simulink model "V90_2MW_TurbineModel_26_11_2021"  (R2020a)
settings: Solver=VariableStepAuto  StartTime=0.0  StopTime=10  RelTol=1e-3  EnableMultiTasking=on
model workspace (MAT data in the model file):
  Tw = Simulink.Parameter
  Tw.Value = [0; 0; 24.07; 18.74; 14.42; 10.93; 8.08; 5.74; 5.8; 4.17; 2.78; 1.59; 0.56; -0.34; -1.13; -1.83; -2.46; -3.02; -3.52; -3.98; -4.39; -3.77; -4.12; -4.43; -4.73]
  Tw.DataType = 'auto'
  Tw.Dimensions = [25 1]
  c = Simulink.Parameter
  c.Value = [3.65; 4.43; 4.56; 4.36; 4.03; 3.68; 3.35; 3.05; 2.79; 2.56; 2.37; 2.19; 2.04; 1.91; 1.79; 1.68; 1.59; 1.5; 1.43; 1.36; 1.29; 1.24; 1.18; 1.14; 1.09]
  c.DataType = 'auto'
  c.Dimensions = [25 1]
  dcm = Simulink.Parameter
  dcm.Value = [0  0  0; 0  0  0; 0  0  0]
  dcm.DataType = 'auto'
  dcm.Dimensions = [3 3]
  r = Simulink.Parameter
  r.Value = [1.8; 3.6; 5.4; 7.2; 9; 10.8; 12.6; 14.4; 16.2; 18; 19.8; 21.6; 23.4; 25.2; 27; 28.8; 30.6; 32.4; 34.2; 36; 37.8; 39.6; 41.4; 43.2; 45]
  r.DataType = 'auto'
  r.Dimensions = [25 1]
values from neighbouring files (symbols this model uses):
  N = 100    [Generator_specs.m]
  s = tf('s')    [Wind_Turbine_Pitch.m]
undefined symbols (not defined in the file or in its folder): T, X, Y, Z
libraries: sm_lib x21, nesl_utility x12, fl_lib x5, aerolibtransform2 x3, aerolibwind2 x3, aerolib6dof2 x1, simulink x1, aerolibasang x1
(part 1 of 2)
settings Model: Creator=Dimple  LastModifiedBy=Dimple
settings DataIOCC: LimitDataPoints=on  MaxDataPoints=10000
settings OptimizationCC: LifeSpan=inf
settings DebuggingCC: AllowSymbolicDim=off  SFUnexpectedBacktrackingDiag=warning  SFNoUnconditionalDefaultTransitionDiag=warning  SFExecutionAtInitializationDiag=none  ArithmeticOperatorsInVariantConditions=warning
settings SFSimCC: SimUseLocalCustomCode=off  CustomCodeUndefinedFunction=UseInterfaceOnly
settings RTWCC: RTWUseLocalCustomCode=off
settings CodeAppCC: StateflowObjectComments=on
settings GRTTargetCC: TargetLangStandard=C89/C90 (ANSI)
settings ConfigComp: CovMetricSettings=dw  CovHtmlReporting=on  CovSaveCumulativeToWorkspaceVar=on  CovSaveSingleToWorkspaceVar=on  CovExternalEMLEnable=off  CovSFcnEnable=off
settings SimscapeCC: SimscapeLogType=all  SimscapeLogSimulationStatistics=on  SimscapeLogDataHistory=10000

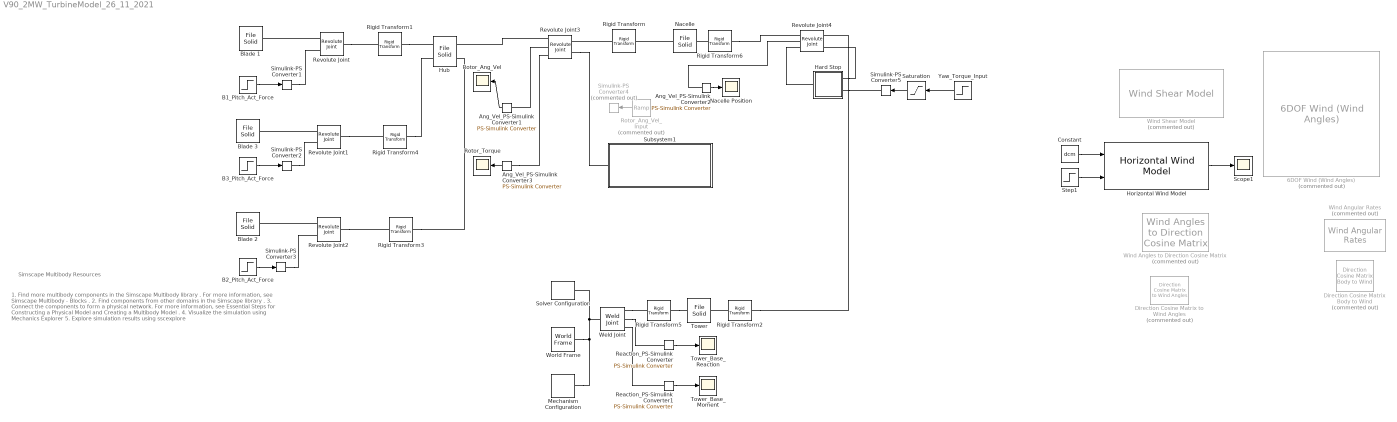
== system V90_2MW_TurbineModel_26_11_2021 ==
  note: 1. Find more multibody components in the Simscape Multibody library .
      | For more information, see Simscape Multibody - Blocks .
      | 2. Find components from other domains in the Simscape library .
      | 3. Connect the components to form a physical network.
      | For more information, see Essential Steps for Constructing a Physical Model and Creating a Multibody Model .
      | 4. Visualize the simulation using Mechanics Explorer
      | 5. Explore simulation results using sscexplore
  note: Simscape Multibody Resources
  6DOF Wind (Wind Angles) : aerolib6dof2/6DOF Wind (Wind Angles)  Commented=on  units=Metric (MKS)  mtype=Fixed  rep=Wind Angles  xme_0=[0 0 0]  Vm_0=[0 0 0]  wind_0=[0 0 0]  pm_0=[0 0 0]  mass_0=1.0  mass_e=0.5  mass_f=2.0  inertia=eye(3)  inertia_e=eye(3)  inertia_f=2*eye(3)  vre_flag=on  abi_flag=off  xme_statename=''  Vm_statename=''  alpha_statename=''  beta_statename=''  wind_statename=''  quat_statename=''  pm_statename=''  mass_statename=''
      settings: SourceProductBaseCode=AE
  Ang_Vel_PS-Simulink Converter1 : nesl_utility/PS-Simulink Converter  PhysicalDomain=network_engine_domain  SubClassName=ps_output  LeftPortType=input  RightPortType=output  PseudoPeriodic=off  Frequencies=[]  Unit=inherit  AffineConversion=off
      settings: SourceProductBaseCode=MT,SS
  Ang_Vel_PS-Simulink Converter2 : nesl_utility/PS-Simulink Converter  PhysicalDomain=network_engine_domain  SubClassName=ps_output  LeftPortType=input  RightPortType=output  PseudoPeriodic=off  Frequencies=[]  Unit=inherit  AffineConversion=off
      settings: SourceProductBaseCode=MT,SS
  Ang_Vel_PS-Simulink Converter3 : nesl_utility/PS-Simulink Converter  PhysicalDomain=network_engine_domain  SubClassName=ps_output  LeftPortType=input  RightPortType=output  PseudoPeriodic=off  Frequencies=[]  Unit=inherit  AffineConversion=off
      settings: SourceProductBaseCode=MT,SS
  B1_Pitch_Act_Force : Step  Time=0.35  After=2  SampleTime=0
  B2_Pitch_Act_Force : Step  Time=0.35  After=2  SampleTime=0
  B3_Pitch_Act_Force : Step  Time=0.35  After=2  SampleTime=0
  Blade 1 : sm_lib/Body Elements/File Solid  ExtGeomFileName=C:\Users\Dimple\Desktop\Dimple\08_ALTRAN\01_Work\Wind Turbine_MBSE Design\01_WT_MBSE\Multibody\WT blade.STEP  UnitType=FromFile  ExtGeomFileUnits=m  StepReaderType=HEX  ExportConvexHullGeometry=off  InertiaType=PointMass  Mass=5388  MassUnits=kg  CenterOfMass=[0 0 0]  CenterOfMassUnits=m  MomentsOfInertia=[1 1 1]  MomentsOfInertiaUnits=kg*m^2  ProductsOfInertia=[0 0 0]  ProductsOfInertiaUnits=kg*m^2  BasedOnType=DensityFromFile  Density=1000  DensityUnits=kg/m^3  DoExposeReferenceFrame=on  SerializedFrames=<Frames/>  GraphicType=FromGeometry  MarkerShape=Sphere  MarkerSize=10  GraphicVisPropType=SimpleVisualProperties  GraphicDiffuseColor=[0.5 0.5 0.5]  GraphicSpecularColor=[0.5 0.5 0.5 1.0]  GraphicAmbientColor=[0.15 0.15 0.15 1.0]  GraphicEmissiveColor=[0.0 0.0 0.0 1.0]  GraphicShininess=75  GraphicOpacity=1.0
  Blade 2 : sm_lib/Body Elements/File Solid  ExtGeomFileName=C:\Users\Dimple\Desktop\Dimple\08_ALTRAN\01_Work\Wind Turbine_MBSE Design\01_WT_MBSE\Multibody\WT blade.STEP  UnitType=FromFile  ExtGeomFileUnits=m  StepReaderType=HEX  ExportConvexHullGeometry=off  InertiaType=PointMass  Mass=5388  MassUnits=kg  CenterOfMass=[0 0 0]  CenterOfMassUnits=m  MomentsOfInertia=[1 1 1]  MomentsOfInertiaUnits=kg*m^2  ProductsOfInertia=[0 0 0]  ProductsOfInertiaUnits=kg*m^2  BasedOnType=DensityFromFile  Density=1000  DensityUnits=kg/m^3  DoExposeReferenceFrame=on  SerializedFrames=<Frames/>  GraphicType=FromGeometry  MarkerShape=Sphere  MarkerSize=10  GraphicVisPropType=SimpleVisualProperties  GraphicDiffuseColor=[0.5 0.5 0.5]  GraphicSpecularColor=[0.5 0.5 0.5 1.0]  GraphicAmbientColor=[0.15 0.15 0.15 1.0]  GraphicEmissiveColor=[0.0 0.0 0.0 1.0]  GraphicShininess=75  GraphicOpacity=1.0
  Blade 3 : sm_lib/Body Elements/File Solid  ExtGeomFileName=C:\Users\Dimple\Desktop\Dimple\08_ALTRAN\01_Work\Wind Turbine_MBSE Design\01_WT_MBSE\Multibody\WT blade.STEP  UnitType=FromFile  ExtGeomFileUnits=m  StepReaderType=HEX  ExportConvexHullGeometry=off  InertiaType=PointMass  Mass=5388  MassUnits=kg  CenterOfMass=[0 0 0]  CenterOfMassUnits=m  MomentsOfInertia=[1 1 1]  MomentsOfInertiaUnits=kg*m^2  ProductsOfInertia=[0 0 0]  ProductsOfInertiaUnits=kg*m^2  BasedOnType=DensityFromFile  Density=1000  DensityUnits=kg/m^3  DoExposeReferenceFrame=on  SerializedFrames=<Frames/>  GraphicType=FromGeometry  MarkerShape=Sphere  MarkerSize=10  GraphicVisPropType=SimpleVisualProperties  GraphicDiffuseColor=[0.5 0.5 0.5]  GraphicSpecularColor=[0.5 0.5 0.5 1.0]  GraphicAmbientColor=[0.15 0.15 0.15 1.0]  GraphicEmissiveColor=[0.0 0.0 0.0 1.0]  GraphicShininess=75  GraphicOpacity=1.0
  Constant : Constant  Value=dcm
  Direction Cosine Matrix Body to Wind : aerolibtransform2/Direction Cosine Matrix Body to Wind  Commented=on
      settings: SourceProductBaseCode=AE
  Direction Cosine Matrix to Wind Angles : aerolibtransform2/Direction Cosine Matrix to Wind Angles  Commented=on  action=None  tolerance=eps(2)
      settings: SourceProductBaseCode=AE
  Hard Stop : Subsystem  mask{ub=pi()/4, lb=0, csub=1e+04, cslb=1e+06, cdub=1e7, cdlb=1e7, iap=0}
      mask prompts: ub "Upper bound (rad)"; lb "Lower bound (rad)"; csub "Contact stiffness at upper bound (N*m/rad)"; cslb "Contact stiffness at lower bound (N*m/rad)"; cdub "Contact damping at upper bound (N*m/(rad/s))"; cdlb "Contact damping at lower bound (N*m/(rad/s))"; iap "Initial angular position"
      mask Display: image(imread('Hard Stop.png'))
  Horizontal Wind Model : aerolibwind2/Horizontal Wind Model  units=Metric (MKS)  Vw_source=External  Vwind=13.5  W_source=Internal  Wdeg=30
      settings: SourceProductBaseCode=AE
  Hub : sm_lib/Body Elements/File Solid  ExtGeomFileName=C:\Users\Dimple\Desktop\Dimple\08_ALTRAN\01_Work\Wind Turbine_MBSE Design\01_WT_MBSE\Multibody\WT hub.STEP  UnitType=FromFile  ExtGeomFileUnits=m  StepReaderType=HEX  ExportConvexHullGeometry=off  InertiaType=PointMass  Mass=18770  MassUnits=kg  CenterOfMass=[0 0 0]  CenterOfMassUnits=m  MomentsOfInertia=[1 1 1]  MomentsOfInertiaUnits=kg*m^2  ProductsOfInertia=[0 0 0]  ProductsOfInertiaUnits=kg*m^2  BasedOnType=DensityFromFile  Density=1000  DensityUnits=kg/m^3  DoExposeReferenceFrame=on  SerializedFrames=<Frames><Frame><Id>Frame1</Id><Value><Name>B1</Name><Origin><Source>GeometricFeature</Source><FeatureName>circular curve 23</FeatureName></Origin><PrimaryAxis><DefinedDirection>+Z</DefinedDirection><Source>ReferenceFrame</Source><SourceDirection>+Y</SourceDirection><FeatureName></FeatureName></PrimaryAxis><SecondaryAxis><DefinedDirection>+X</DefinedDirection><Source>ReferenceFrame</Source><SourceDirection>+X</SourceDirection><FeatureName></FeatureName></SecondaryAxis></Value></Frame><Frame><Id>Frame3</Id><Value><Name>B3</Name><Origin><Source>GeometricFeature</Source><FeatureName>circular curve 21</FeatureName></Origin><PrimaryAxis><DefinedDirection>+Z</DefinedDirection><Source>ReferenceFrame</Source><SourceDirection>-X</SourceDirection><FeatureName></FeatureName></PrimaryAxis><SecondaryAxis><DefinedDirection>+X</DefinedDirection><Source>ReferenceFrame</Source><SourceDirection>-Y</SourceDirection><FeatureName></FeatureName></SecondaryAxis></Value></Frame><Frame><Id>Frame4</Id><Value><Name>B2</Name><Origin><Source>GeometricFeature</Source><FeatureName>circular curve 25</FeatureName></Origin><PrimaryAxis><DefinedDirection>+Z</DefinedDirection><Source>ReferenceFrame</Source><SourceDirection>+X</SourceDirection><FeatureName></FeatureName></PrimaryAxis><SecondaryAxis><DefinedDirection>+X</DefinedDirection><Source>ReferenceFrame</Source><SourceDirection>+Y</SourceDirection><FeatureName></FeatureName></SecondaryAxis></Value></Frame></Frames>  GraphicType=FromGeometry  MarkerShape=Sphere  MarkerSize=10  GraphicVisPropType=SimpleVisualProperties  GraphicDiffuseColor=[0.5 0.5 0.5]  GraphicSpecularColor=[0.5 0.5 0.5 1.0]  GraphicAmbientColor=[0.15 0.15 0.15 1.0]  GraphicEmissiveColor=[0.0 0.0 0.0 1.0]  GraphicShininess=75  GraphicOpacity=1.0
  Mechanism Configuration : sm_lib/Utilities/Mechanism Configuration  UniformGravity=Constant  GravityVector=[0 -9.80665 0]  GravityUnits=m/s^2  LinearizationDelta=0.001
  Nacelle : sm_lib/Body Elements/File Solid  ExtGeomFileName=C:\Users\Dimple\Desktop\Dimple\08_ALTRAN\01_Work\Wind Turbine_MBSE Design\01_WT_MBSE\Multibody\WT nacelle.STEP  UnitType=FromFile  ExtGeomFileUnits=m  StepReaderType=HEX  ExportConvexHullGeometry=off  InertiaType=PointMass  Mass=56310  MassUnits=kg  CenterOfMass=[0 0 0]  CenterOfMassUnits=m  MomentsOfInertia=[1 1 1]  MomentsOfInertiaUnits=kg*m^2  ProductsOfInertia=[0 0 0]  ProductsOfInertiaUnits=kg*m^2  BasedOnType=DensityFromFile  Density=1000  DensityUnits=kg/m^3  DoExposeReferenceFrame=on  SerializedFrames=<Frames><Frame><Id>Frame1</Id><Value><Name>T</Name><Origin><Source>GeometricFeature</Source><FeatureName>circular curve 2</FeatureName></Origin><PrimaryAxis><DefinedDirection>+Z</DefinedDirection><Source>ReferenceFrame</Source><SourceDirection>+Z</SourceDirection><FeatureName></FeatureName></PrimaryAxis><SecondaryAxis><DefinedDirection>+X</DefinedDirection><Source>ReferenceFrame</Source><SourceDirection>+X</SourceDirection><FeatureName></FeatureName></SecondaryAxis></Value></Frame></Frames>  GraphicType=FromGeometry  MarkerShape=Sphere  MarkerSize=10  GraphicVisPropType=SimpleVisualProperties  GraphicDiffuseColor=[0.5 0.5 0.5]  GraphicSpecularColor=[0.5 0.5 0.5 1.0]  GraphicAmbientColor=[0.15 0.15 0.15 1.0]  GraphicEmissiveColor=[0.0 0.0 0.0 1.0]  GraphicShininess=75  GraphicOpacity=1.0
  Nacelle Position : Scope
  Reaction_PS-Simulink Converter : nesl_utility/PS-Simulink Converter  PhysicalDomain=network_engine_domain  SubClassName=ps_output  LeftPortType=input  RightPortType=output  PseudoPeriodic=off  Frequencies=[]  Unit=inherit  AffineConversion=off
      settings: SourceProductBaseCode=MT,SS
  Reaction_PS-Simulink Converter1 : nesl_utility/PS-Simulink Converter  PhysicalDomain=network_engine_domain  SubClassName=ps_output  LeftPortType=input  RightPortType=output  PseudoPeriodic=off  Frequencies=[]  Unit=inherit  AffineConversion=off
      settings: SourceProductBaseCode=MT,SS
  Revolute Joint : sm_lib/Joints/Revolute Joint  JointMode=Normal  SenseConstraintForce=off  SenseConstraintForceX=off  SenseConstraintForceY=off  SenseConstraintForceZ=off  SenseConstraintTorque=off  SenseConstraintTorqueX=off  SenseConstraintTorqueY=off  SenseConstraintTorqueZ=off  SenseTotalForce=off  SenseTotalForceX=off  SenseTotalForceY=off  SenseTotalForceZ=off  SenseTotalTorque=off  SenseTotalTorqueX=off  SenseTotalTorqueY=off  SenseTotalTorqueZ=off  CompositeWrenchDir=BaseOnFollower  CompositeWrenchFrame=BaseFrame  EquilibriumPosition=0  EquilibriumPositionUnits=deg  SpringStiffness=0  SpringStiffnessUnits=N*m/deg  DampingCoefficient=0  DampingCoefficientUnits=N*m/(deg/s)  TorqueActuationMode=ComputedTorque  MotionActuationMode=InputMotion  SensePosition=off  SenseVelocity=off  SenseAcceleration=off  SenseTorqueForce=off  SenseLowerLimitTorqueForce=off  SenseUpperLimitTorqueForce=off  LowerLimitSpecify=off  LowerLimitBound=-90  LowerLimitBoundUnits=deg  LowerLimitStiffness=1e4  LowerLimitStiffnessUnits=N*m/deg  LowerLimitDamping=10  LowerLimitDampingUnits=N*m/(deg/s)  LowerLimitTransitionRegionWidth=0.1  LowerLimitTransitionRegionWidthUnits=deg  UpperLimitSpecify=off  UpperLimitBound=90  UpperLimitBoundUnits=deg  UpperLimitStiffness=1e4  UpperLimitStiffnessUnits=N*m/deg  UpperLimitDamping=10  UpperLimitDampingUnits=N*m/(deg/s)  UpperLimitTransitionRegionWidth=0.1  UpperLimitTransitionRegionWidthUnits=deg  PositionTargetSpecify=off  PositionTargetPriority=High  PositionTargetValue=30  PositionTargetValueUnits=deg  VelocityTargetSpecify=off  VelocityTargetPriority=High  VelocityTargetValue=0  VelocityTargetValueUnits=deg/s
  Revolute Joint1 : sm_lib/Joints/Revolute Joint  JointMode=Normal  SenseConstraintForce=off  SenseConstraintForceX=off  SenseConstraintForceY=off  SenseConstraintForceZ=off  SenseConstraintTorque=off  SenseConstraintTorqueX=off  SenseConstraintTorqueY=off  SenseConstraintTorqueZ=off  SenseTotalForce=off  SenseTotalForceX=off  SenseTotalForceY=off  SenseTotalForceZ=off  SenseTotalTorque=off  SenseTotalTorqueX=off  SenseTotalTorqueY=off  SenseTotalTorqueZ=off  CompositeWrenchDir=BaseOnFollower  CompositeWrenchFrame=BaseFrame  EquilibriumPosition=0  EquilibriumPositionUnits=deg  SpringStiffness=0  SpringStiffnessUnits=N*m/deg  DampingCoefficient=0  DampingCoefficientUnits=N*m/(deg/s)  TorqueActuationMode=ComputedTorque  MotionActuationMode=InputMotion  SensePosition=off  SenseVelocity=off  SenseAcceleration=off  SenseTorqueForce=off  SenseLowerLimitTorqueForce=off  SenseUpperLimitTorqueForce=off  LowerLimitSpecify=off  LowerLimitBound=-90  LowerLimitBoundUnits=deg  LowerLimitStiffness=1e4  LowerLimitStiffnessUnits=N*m/deg  LowerLimitDamping=10  LowerLimitDampingUnits=N*m/(deg/s)  LowerLimitTransitionRegionWidth=0.1  LowerLimitTransitionRegionWidthUnits=deg  UpperLimitSpecify=off  UpperLimitBound=90  UpperLimitBoundUnits=deg  UpperLimitStiffness=1e4  UpperLimitStiffnessUnits=N*m/deg  UpperLimitDamping=10  UpperLimitDampingUnits=N*m/(deg/s)  UpperLimitTransitionRegionWidth=0.1  UpperLimitTransitionRegionWidthUnits=deg  PositionTargetSpecify=off  PositionTargetPriority=High  PositionTargetValue=30  PositionTargetValueUnits=deg  VelocityTargetSpecify=off  VelocityTargetPriority=High  VelocityTargetValue=0  VelocityTargetValueUnits=deg/s
  Revolute Joint2 : sm_lib/Joints/Revolute Joint  JointMode=Normal  SenseConstraintForce=off  SenseConstraintForceX=off  SenseConstraintForceY=off  SenseConstraintForceZ=off  SenseConstraintTorque=off  SenseConstraintTorqueX=off  SenseConstraintTorqueY=off  SenseConstraintTorqueZ=off  SenseTotalForce=off  SenseTotalForceX=off  SenseTotalForceY=off  SenseTotalForceZ=off  SenseTotalTorque=off  SenseTotalTorqueX=off  SenseTotalTorqueY=off  SenseTotalTorqueZ=off  CompositeWrenchDir=BaseOnFollower  CompositeWrenchFrame=BaseFrame  EquilibriumPosition=0  EquilibriumPositionUnits=deg  SpringStiffness=0  SpringStiffnessUnits=N*m/deg  DampingCoefficient=0  DampingCoefficientUnits=N*m/(deg/s)  TorqueActuationMode=ComputedTorque  MotionActuationMode=InputMotion  SensePosition=off  SenseVelocity=off  SenseAcceleration=off  SenseTorqueForce=off  SenseLowerLimitTorqueForce=off  SenseUpperLimitTorqueForce=off  LowerLimitSpecify=off  LowerLimitBound=-90  LowerLimitBoundUnits=deg  LowerLimitStiffness=1e4  LowerLimitStiffnessUnits=N*m/deg  LowerLimitDamping=10  LowerLimitDampingUnits=N*m/(deg/s)  LowerLimitTransitionRegionWidth=0.1  LowerLimitTransitionRegionWidthUnits=deg  UpperLimitSpecify=off  UpperLimitBound=90  UpperLimitBoundUnits=deg  UpperLimitStiffness=1e4  UpperLimitStiffnessUnits=N*m/deg  UpperLimitDamping=10  UpperLimitDampingUnits=N*m/(deg/s)  UpperLimitTransitionRegionWidth=0.1  UpperLimitTransitionRegionWidthUnits=deg  PositionTargetSpecify=off  PositionTargetPriority=High  PositionTargetValue=30  PositionTargetValueUnits=deg  VelocityTargetSpecify=off  VelocityTargetPriority=High  VelocityTargetValue=0  VelocityTargetValueUnits=deg/s
  Revolute Joint3 : sm_lib/Joints/Revolute Joint  JointMode=Normal  SenseConstraintForce=off  SenseConstraintForceX=off  SenseConstraintForceY=off  SenseConstraintForceZ=off  SenseConstraintTorque=off  SenseConstraintTorqueX=off  SenseConstraintTorqueY=off  SenseConstraintTorqueZ=off  SenseTotalForce=off  SenseTotalForceX=off  SenseTotalForceY=off  SenseTotalForceZ=off  SenseTotalTorque=off  SenseTotalTorqueX=off  SenseTotalTorqueY=off  SenseTotalTorqueZ=off  CompositeWrenchDir=FollowerOnBase  CompositeWrenchFrame=BaseFrame  EquilibriumPosition=0  EquilibriumPositionUnits=deg  SpringStiffness=0  SpringStiffnessUnits=N*m/deg  DampingCoefficient=0  DampingCoefficientUnits=N*m/(deg/s)  TorqueActuationMode=InputTorque  MotionActuationMode=ComputedMotion  SensePosition=off  SenseVelocity=on  SenseAcceleration=off  SenseTorqueForce=on  SenseLowerLimitTorqueForce=off  SenseUpperLimitTorqueForce=off  LowerLimitSpecify=off  LowerLimitBound=-90  LowerLimitBoundUnits=deg  LowerLimitStiffness=1e4  LowerLimitStiffnessUnits=N*m/deg  LowerLimitDamping=10  LowerLimitDampingUnits=N*m/(deg/s)  LowerLimitTransitionRegionWidth=0.1  LowerLimitTransitionRegionWidthUnits=deg  UpperLimitSpecify=off  UpperLimitBound=90  UpperLimitBoundUnits=deg  UpperLimitStiffness=1e4  UpperLimitStiffnessUnits=N*m/deg  UpperLimitDamping=10  UpperLimitDampingUnits=N*m/(deg/s)  UpperLimitTransitionRegionWidth=0.1  UpperLimitTransitionRegionWidthUnits=deg  PositionTargetSpecify=off  PositionTargetPriority=High  PositionTargetValue=0  PositionTargetValueUnits=deg  VelocityTargetSpecify=off  VelocityTargetPriority=High  VelocityTargetValue=0  VelocityTargetValueUnits=deg/s
  Revolute Joint4 : sm_lib/Joints/Revolute Joint  JointMode=Normal  SenseConstraintForce=off  SenseConstraintForceX=off  SenseConstraintForceY=off  SenseConstraintForceZ=off  SenseConstraintTorque=off  SenseConstraintTorqueX=off  SenseConstraintTorqueY=off  SenseConstraintTorqueZ=off  SenseTotalForce=off  SenseTotalForceX=off  SenseTotalForceY=off  SenseTotalForceZ=off  SenseTotalTorque=off  SenseTotalTorqueX=off  SenseTotalTorqueY=off  SenseTotalTorqueZ=off  CompositeWrenchDir=FollowerOnBase  CompositeWrenchFrame=BaseFrame  EquilibriumPosition=0  EquilibriumPositionUnits=deg  SpringStiffness=0  SpringStiffnessUnits=N*m/deg  DampingCoefficient=0  DampingCoefficientUnits=N*m/(deg/s)  TorqueActuationMode=InputTorque  MotionActuationMode=ComputedMotion  SensePosition=on  SenseVelocity=on  SenseAcceleration=off  SenseTorqueForce=off  SenseLowerLimitTorqueForce=off  SenseUpperLimitTorqueForce=off  LowerLimitSpecify=off  LowerLimitBound=0  LowerLimitBoundUnits=deg  LowerLimitStiffness=1e4  LowerLimitStiffnessUnits=N*m/deg  LowerLimitDamping=10  LowerLimitDampingUnits=N*m/(deg/s)  LowerLimitTransitionRegionWidth=0.1  LowerLimitTransitionRegionWidthUnits=deg  UpperLimitSpecify=off  UpperLimitBound=120  UpperLimitBoundUnits=deg  UpperLimitStiffness=1e4  UpperLimitStiffnessUnits=N*m/deg  UpperLimitDamping=10  UpperLimitDampingUnits=N*m/(deg/s)  UpperLimitTransitionRegionWidth=0.1  UpperLimitTransitionRegionWidthUnits=deg  PositionTargetSpecify=off  PositionTargetPriority=High  PositionTargetValue=30  PositionTargetValueUnits=deg  VelocityTargetSpecify=off  VelocityTargetPriority=High  VelocityTargetValue=0  VelocityTargetValueUnits=deg/s
  Rigid Transform : sm_lib/Frames and Transforms/Rigid Transform  TranslationMethod=StandardAxis  TranslationStandardOffset=4.5  TranslationLengthUnit=m  TranslationStandardAxis=+Z  TranslationCartesianOffset=[0 0 0]  TranslationROffset=0  TranslationROffsetUnits=m  TranslationZOffset=0  TranslationZOffsetUnits=m  TranslationThetaOffset=0  TranslationThetaOffsetUnits=deg  RotationMethod=None  RotationAngleUnits=deg  RotationStandardAxis=+Z  RotationAngle=0.0  RotationArbitraryAxis=[0 0 1]  FollAlignAxisA=+X  BaseAlignAxisA=+Y  FollAlignAxisB=+Y  BaseAlignAxisB=+Z  RotationSequenceAxes=FollowerAxes  RotationSequence=XYX  RotationSequenceAngles=[0 0 0]  RotationSequenceAnglesUnits=deg  RotationMatrix=[1 0 0; 0 1 0; 0 0 1]
  Rigid Transform1 : sm_lib/Frames and Transforms/Rigid Transform  TranslationMethod=StandardAxis  TranslationStandardOffset=3.5  TranslationLengthUnit=m  TranslationStandardAxis=+Z  TranslationCartesianOffset=[0 0 0]  TranslationROffset=0  TranslationROffsetUnits=m  TranslationZOffset=0  TranslationZOffsetUnits=m  TranslationThetaOffset=0  TranslationThetaOffsetUnits=deg  RotationMethod=StandardAxis  RotationAngleUnits=deg  RotationStandardAxis=+Z  RotationAngle=180  RotationArbitraryAxis=[0 0 1]  FollAlignAxisA=+X  BaseAlignAxisA=+Y  FollAlignAxisB=+Y  BaseAlignAxisB=+Z  RotationSequenceAxes=FollowerAxes  RotationSequence=XYX  RotationSequenceAngles=[0 0 0]  RotationSequenceAnglesUnits=deg  RotationMatrix=[1 0 0; 0 1 0; 0 0 1]
  Rigid Transform2 : sm_lib/Frames and Transforms/Rigid Transform  TranslationMethod=None  TranslationStandardOffset=4.5  TranslationLengthUnit=m  TranslationStandardAxis=-Z  TranslationCartesianOffset=[0 0 0]  TranslationROffset=0  TranslationROffsetUnits=m  TranslationZOffset=0  TranslationZOffsetUnits=m  TranslationThetaOffset=0  TranslationThetaOffsetUnits=deg  RotationMethod=AlignedAxes  RotationAngleUnits=deg  RotationStandardAxis=+Z  RotationAngle=0.0  RotationArbitraryAxis=[0 0 1]  FollAlignAxisA=+Z  BaseAlignAxisA=+Y  FollAlignAxisB=+X  BaseAlignAxisB=+X  RotationSequenceAxes=FollowerAxes  RotationSequence=XYX  RotationSequenceAngles=[0 0 0]  RotationSequenceAnglesUnits=deg  RotationMatrix=[1 0 0; 0 1 0; 0 0 1]
  Rigid Transform3 : sm_lib/Frames and Transforms/Rigid Transform  TranslationMethod=StandardAxis  TranslationStandardOffset=3.5  TranslationLengthUnit=m  TranslationStandardAxis=-Z  TranslationCartesianOffset=[0 0 0]  TranslationROffset=0  TranslationROffsetUnits=m  TranslationZOffset=0  TranslationZOffsetUnits=m  TranslationThetaOffset=0  TranslationThetaOffsetUnits=deg  RotationMethod=StandardAxis  RotationAngleUnits=deg  RotationStandardAxis=+Y  RotationAngle=30  RotationArbitraryAxis=[0 0 1]  FollAlignAxisA=+X  BaseAlignAxisA=+Y  FollAlignAxisB=+Y  BaseAlignAxisB=+Z  RotationSequenceAxes=FollowerAxes  RotationSequence=XYX  RotationSequenceAngles=[0 0 0]  RotationSequenceAnglesUnits=deg  RotationMatrix=[1 0 0; 0 1 0; 0 0 1]
  Rigid Transform4 : sm_lib/Frames and Transforms/Rigid Transform  TranslationMethod=StandardAxis  TranslationStandardOffset=3.5  TranslationLengthUnit=m  TranslationStandardAxis=-Z  TranslationCartesianOffset=[0 0 0]  TranslationROffset=0  TranslationROffsetUnits=m  TranslationZOffset=0  TranslationZOffsetUnits=m  TranslationThetaOffset=0  TranslationThetaOffsetUnits=deg  RotationMethod=StandardAxis  RotationAngleUnits=deg  RotationStandardAxis=-Y  RotationAngle=30  RotationArbitraryAxis=[0 0 1]  FollAlignAxisA=+X  BaseAlignAxisA=+Y  FollAlignAxisB=+Y  BaseAlignAxisB=+Z  RotationSequenceAxes=FollowerAxes  RotationSequence=XYX  RotationSequenceAngles=[0 0 0]  RotationSequenceAnglesUnits=deg  RotationMatrix=[1 0 0; 0 1 0; 0 0 1]
  Rigid Transform5 : sm_lib/Frames and Transforms/Rigid Transform  TranslationMethod=None  TranslationStandardOffset=4.5  TranslationLengthUnit=m  TranslationStandardAxis=-Z  TranslationCartesianOffset=[0 0 0]  TranslationROffset=0  TranslationROffsetUnits=m  TranslationZOffset=0  TranslationZOffsetUnits=m  TranslationThetaOffset=0  TranslationThetaOffsetUnits=deg  RotationMethod=None  RotationAngleUnits=deg  RotationStandardAxis=+Z  RotationAngle=0.0  RotationArbitraryAxis=[0 0 1]  FollAlignAxisA=+X  BaseAlignAxisA=+Y  FollAlignAxisB=+Y  BaseAlignAxisB=+Z  RotationSequenceAxes=FollowerAxes  RotationSequence=XYX  RotationSequenceAngles=[0 0 0]  RotationSequenceAnglesUnits=deg  RotationMatrix=[1 0 0; 0 1 0; 0 0 1]
  Rigid Transform6 : sm_lib/Frames and Transforms/Rigid Transform  TranslationMethod=None  TranslationStandardOffset=4.5  TranslationLengthUnit=m  TranslationStandardAxis=-Z  TranslationCartesianOffset=[0 0 0]  TranslationROffset=0  TranslationROffsetUnits=m  TranslationZOffset=0  TranslationZOffsetUnits=m  TranslationThetaOffset=0  TranslationThetaOffsetUnits=deg  RotationMethod=AlignedAxes  RotationAngleUnits=deg  RotationStandardAxis=+Z  RotationAngle=0.0  RotationArbitraryAxis=[0 0 1]  FollAlignAxisA=+Z  BaseAlignAxisA=+Y  FollAlignAxisB=+X  BaseAlignAxisB=+X  RotationSequenceAxes=FollowerAxes  RotationSequence=XYX  RotationSequenceAngles=[0 0 0]  RotationSequenceAnglesUnits=deg  RotationMatrix=[1 0 0; 0 1 0; 0 0 1]
  Rotor_Ang_Vel : Scope
  Rotor_Ang_Vel_Input : simulink/Sources/Ramp  Commented=on  slope=1.56  start=1  InitialOutput=0
  Rotor_Torque : Scope
  Saturation : Saturate  UpperLimit=1e8  LowerLimit=1e-8
  Scope1 : Scope
  Simulink-PS Converter1 : nesl_utility/Simulink-PS Converter  PhysicalDomain=network_engine_domain  SubClassName=ps_input  LeftPortType=input  RightPortType=output  PseudoPeriodic=off  Frequencies=[]  NoiseDistribution=none  NoiseParameters=[]  Unit=1  AffineConversion=off  FilteringAndDerivatives=filter  SimscapeFilterOrder=2  InputFilterTimeConstant=0.001  UdotUserProvided=0
      settings: SourceProductBaseCode=MT,SS
  Simulink-PS Converter2 : nesl_utility/Simulink-PS Converter  PhysicalDomain=network_engine_domain  SubClassName=ps_input  LeftPortType=input  RightPortType=output  PseudoPeriodic=off  Frequencies=[]  NoiseDistribution=none  NoiseParameters=[]  Unit=1  AffineConversion=off  FilteringAndDerivatives=filter  SimscapeFilterOrder=2  InputFilterTimeConstant=0.001  UdotUserProvided=0
      settings: SourceProductBaseCode=MT,SS
  Simulink-PS Converter3 : nesl_utility/Simulink-PS Converter  PhysicalDomain=network_engine_domain  SubClassName=ps_input  LeftPortType=input  RightPortType=output  PseudoPeriodic=off  Frequencies=[]  NoiseDistribution=none  NoiseParameters=[]  Unit=1  AffineConversion=off  FilteringAndDerivatives=filter  SimscapeFilterOrder=2  InputFilterTimeConstant=0.001  UdotUserProvided=0
      settings: SourceProductBaseCode=MT,SS
  Simulink-PS Converter4 : nesl_utility/Simulink-PS Converter  Commented=on  PhysicalDomain=network_engine_domain  SubClassName=ps_input  LeftPortType=input  RightPortType=output  PseudoPeriodic=off  Frequencies=[]  NoiseDistribution=none  NoiseParameters=[]  Unit=1  AffineConversion=off  FilteringAndDerivatives=filter  SimscapeFilterOrder=2  InputFilterTimeConstant=0.001  UdotUserProvided=0
      settings: SourceProductBaseCode=MT,SS
  Simulink-PS Converter5 : nesl_utility/Simulink-PS Converter  PhysicalDomain=network_engine_domain  SubClassName=ps_input  LeftPortType=input  RightPortType=output  PseudoPeriodic=off  Frequencies=[]  NoiseDistribution=none  NoiseParameters=[]  Unit=1  AffineConversion=off  FilteringAndDerivatives=provide  SimscapeFilterOrder=1  InputFilterTimeConstant=0.001  UdotUserProvided=0
      settings: SourceProductBaseCode=MT,SS
  Solver Configuration : nesl_utility/Solver Configuration  PhysicalDomain=network_engine_domain  SubClassName=solver  LeftPortType=input  RightPortType=generic  Tones=[]  Harmonics=[]  SimulateNoise=off  Profile=off  UseLocalSampling=off  EnableSwitchedLinearOptims=on  FrequencyDomain=off  UseCCode=off  RelTol=0.001  AbsTol=1e-06  MinStep=1e-09  ToWorkspace=off  RevertToSquareIcSolve=off  NumHomotopyIterations=100  PhasorMode=off  PhasorModeNumHarmonics=1  DoDC=off  ResidualTolerance=1e-09  UseLocalSolver=off  LocalSolverChoice=NE_BACKWARD_EULER_ADVANCER  LocalSolverSampleTime=0.001  DoFixedCost=off  MaxNonlinIter=3  MaxModeIter=2  LinearAlgebra=Sparse  EquationFormulation=NE_TIME_EF  DelaysMemoryBudget=1024  AutomaticFiltering=on  FilteringTimeConstant=0.001  PartitionStorageMethod=AS_NEEDED  PartitionMemoryBudget=1024  PartitionMethod=FAST
      settings: SourceProductBaseCode=MT,SS
  Step1 : Step  Time=0  After=13.5  SampleTime=0
  Subsystem1 : Subsystem
  Tower : sm_lib/Body Elements/File Solid  ExtGeomFileName=C:\Users\Dimple\Desktop\Dimple\08_ALTRAN\01_Work\Wind Turbine_MBSE Design\01_WT_MBSE\Multibody\WT tower.STEP  UnitType=FromFile  ExtGeomFileUnits=m  StepReaderType=HEX  ExportConvexHullGeometry=off  InertiaType=PointMass  Mass=115614.8  MassUnits=kg  CenterOfMass=[0 0 0]  CenterOfMassUnits=m  MomentsOfInertia=[1 1 1]  MomentsOfInertiaUnits=kg*m^2  ProductsOfInertia=[0 0 0]  ProductsOfInertiaUnits=kg*m^2  BasedOnType=DensityFromFile  Density=1000  DensityUnits=kg/m^3  DoExposeReferenceFrame=on  SerializedFrames=<Frames><Frame><Id>Frame1</Id><Value><Name>F1</Name><Origin><Source>GeometricFeature</Source><FeatureName>circular curve 3</FeatureName></Origin><PrimaryAxis><DefinedDirection>+Y</DefinedDirection><Source>ReferenceFrame</Source><SourceDirection>+Y</SourceDirection><FeatureName></FeatureName></PrimaryAxis><SecondaryAxis><DefinedDirection>+X</DefinedDirection><Source>ReferenceFrame</Source><SourceDirection>+X</SourceDirection><FeatureName></FeatureName></SecondaryAxis></Value></Frame></Frames>  GraphicType=FromGeometry  MarkerShape=Sphere  MarkerSize=10  GraphicVisPropType=SimpleVisualProperties  GraphicDiffuseColor=[0.5 0.5 0.5]  GraphicSpecularColor=[0.5 0.5 0.5 1.0]  GraphicAmbientColor=[0.15 0.15 0.15 1.0]  GraphicEmissiveColor=[0.0 0.0 0.0 1.0]  GraphicShininess=75  GraphicOpacity=1.0
  Tower_Base_Moment : Scope
  Tower_Base_Reaction : Scope
  Weld Joint : sm_lib/Joints/Weld Joint  JointMode=Normal  SenseConstraintForce=off  SenseConstraintForceX=off  SenseConstraintForceY=off  SenseConstraintForceZ=off  SenseConstraintTorque=off  SenseConstraintTorqueX=off  SenseConstraintTorqueY=off  SenseConstraintTorqueZ=off  SenseTotalForce=on  SenseTotalForceX=off  SenseTotalForceY=off  SenseTotalForceZ=off  SenseTotalTorque=on  SenseTotalTorqueX=off  SenseTotalTorqueY=off  SenseTotalTorqueZ=off  CompositeWrenchDir=FollowerOnBase  CompositeWrenchFrame=BaseFrame
  Wind Angles to Direction Cosine Matrix : aerolibtransform2/Wind Angles to  Direction Cosine Matrix  Commented=on
      settings: SourceProductBaseCode=AE
  Wind Angular Rates : aerolibasang/Wind Angular Rates  Commented=on
      settings: SourceProductBaseCode=AE
  Wind Shear Model : aerolibwind2/Wind Shear Model  Commented=on  units=Metric (MKS)  phase=Category C - Terminal Flight Phase  W_20=15  Wdeg=0
  World Frame : sm_lib/Frames and Transforms/World Frame
  Yaw_Torque_Input : Step  Time=5  After=303000  SampleTime=0
  wires:
  Reaction_PS-Simulink Converter/1 -> Tower_Base_Reaction/1
  B1_Pitch_Act_Force/1 -> Simulink-PS Converter1/1
  B3_Pitch_Act_Force/1 -> Simulink-PS Converter2/1
  B2_Pitch_Act_Force/1 -> Simulink-PS Converter3/1
  Rotor_Ang_Vel_Input/1 -> Simulink-PS Converter4/1
  Ang_Vel_PS-Simulink Converter1/1 -> Rotor_Ang_Vel/1
  Reaction_PS-Simulink Converter1/1 -> Tower_Base_Moment/1
  Constant/1 -> Horizontal Wind Model/1
  Horizontal Wind Model/1 -> Scope1/1
  Yaw_Torque_Input/1 -> Saturation/1
  Step1/1 -> Horizontal Wind Model/2
  Saturation/1 -> Simulink-PS Converter5/1
  Ang_Vel_PS-Simulink Converter2/1 -> Nacelle Position/1
  Ang_Vel_PS-Simulink Converter3/1 -> Rotor_Torque/1
  connections:
  Mechanism Configuration/RConn1 -- Solver Configuration/RConn1 -- Weld Joint/LConn1 -- World Frame/RConn1
  Rigid Transform5/RConn1 -- Tower/LConn1
  Nacelle/RConn1 -- Rigid Transform/LConn1
  Rigid Transform/RConn1 -- Revolute Joint3/LConn1
  Revolute Joint3/RConn1 -- Hub/RConn1
  Rigid Transform1/LConn1 -- Hub/LConn1
  Rigid Transform4/RConn1 -- Hub/LConn2
  Rigid Transform3/RConn1 -- Hub/RConn2
  Revolute Joint/LConn1 -- Blade 1/RConn1
  Revolute Joint/RConn1 -- Rigid Transform1/RConn1
  Simulink-PS Converter1/RConn1 -- Revolute Joint/LConn2
  Revolute Joint1/RConn1 -- Rigid Transform4/LConn1
  Revolute Joint1/LConn1 -- Blade 3/RConn1
  Simulink-PS Converter2/RConn1 -- Revolute Joint1/LConn2
  Revolute Joint2/LConn1 -- Blade 2/RConn1
  Revolute Joint2/RConn1 -- Rigid Transform3/LConn1
  Simulink-PS Converter3/RConn1 -- Revolute Joint2/LConn2
  Weld Joint/RConn1 -- Rigid Transform5/LConn1
  Weld Joint/RConn2 -- Reaction_PS-Simulink Converter/LConn1
  Revolute Joint3/RConn2 -- Ang_Vel_PS-Simulink Converter1/LConn1
  Rigid Transform2/LConn1 -- Tower/RConn1
  Rigid Transform2/RConn1 -- Revolute Joint4/LConn1
  Rigid Transform6/RConn1 -- Revolute Joint4/RConn1
  Rigid Transform6/LConn1 -- Nacelle/LConn1
  Weld Joint/RConn3 -- Reaction_PS-Simulink Converter1/LConn1
  Hard Stop/LConn2 -- Simulink-PS Converter5/RConn1
  Hard Stop/LConn1 -- Revolute Joint4/LConn2
  Revolute Joint4/RConn3 -- Hard Stop/RConn1
  Ang_Vel_PS-Simulink Converter2/LConn1 -- Revolute Joint4/RConn2
  Revolute Joint3/LConn2 -- Subsystem1/RConn1
  Ang_Vel_PS-Simulink Converter3/LConn1 -- Revolute Joint3/RConn3

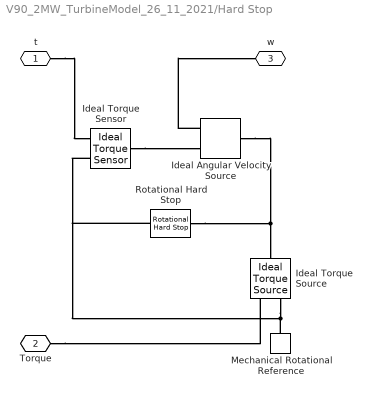
== system V90_2MW_TurbineModel_26_11_2021/Hard Stop ==
  Ideal Angular Velocity Source : fl_lib/Mechanical/Mechanical Sources/Ideal Angular Velocity Source
  Ideal Torque Sensor : fl_lib/Mechanical/Mechanical Sensors/Ideal Torque Sensor
  Ideal Torque Source : fl_lib/Mechanical/Mechanical Sources/Ideal Torque Source
  Mechanical Rotational Reference : fl_lib/Mechanical/Rotational Elements/Mechanical Rotational Reference
  Rotational Hard Stop : fl_lib/Mechanical/Rotational Elements/Rotational Hard Stop  upper_bnd=ub rad  lower_bnd=lb rad  stiff_up=csub N*m/rad  stiff_low=cslb N*m/rad  D_up=cdub N*m/(rad/s)  D_low=cdlb N*m/(rad/s)  model=3  transition=0.001 rad  w_specify=off  w_priority=None  w=0 rad/s  w_nominal_specify=off  w_nominal_unit=rad/s  w_nominal_value=1  t_specify=off  t_priority=None  t=0 N*m  t_nominal_specify=off  t_nominal_unit=N*m  t_nominal_value=1  phi_specify=on  phi_priority=High  phi=iap rad  phi_nominal_specify=off  phi_nominal_unit=rad  phi_nominal_value=1
      settings: SourceProductBaseCode=SS
  t : PMIOPort  Side=Left
  Torque : PMIOPort  Port=2  Side=Left
  w : PMIOPort  Port=3  Side=Right
  connections:
  Mechanical Rotational Reference/LConn1 -- Rotational Hard Stop/RConn1 -- Ideal Torque Sensor/RConn1 -- Ideal Torque Source/RConn2
  Torque/RConn1 -- Ideal Torque Source/RConn1
  Rotational Hard Stop/LConn1 -- Ideal Torque Source/LConn1 -- Ideal Angular Velocity Source/LConn1
  t/RConn1 -- Ideal Torque Sensor/RConn2
  Ideal Torque Sensor/LConn1 -- Ideal Angular Velocity Source/RConn2
  Ideal Angular Velocity Source/RConn1 -- w/RConn1

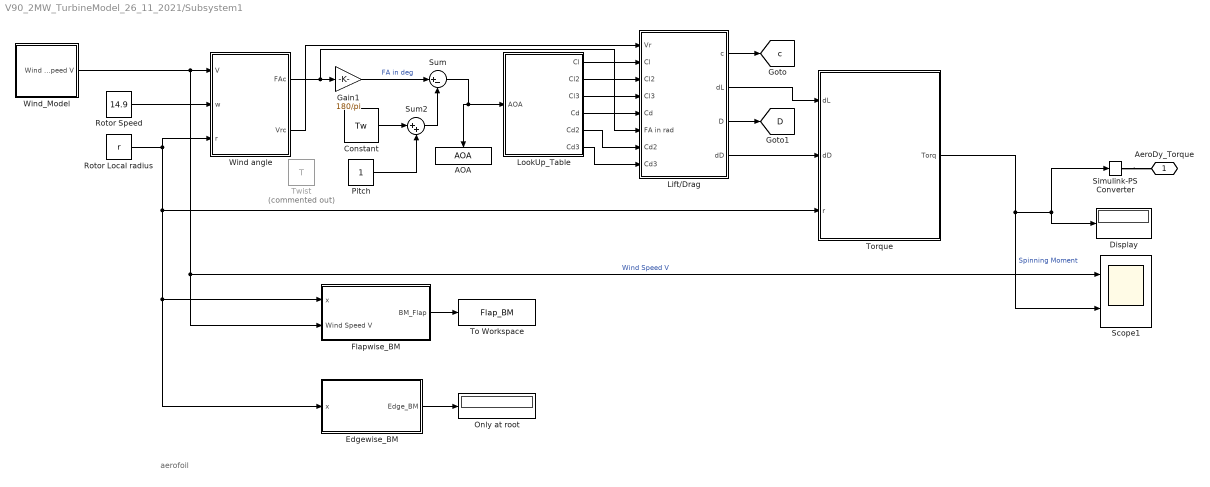
== system V90_2MW_TurbineModel_26_11_2021/Subsystem1 ==
  note: aerofoil
  AOA : ToWorkspace  VariableName=AOA  SampleTime=-1
      settings: Save2DSignal=2-D array (concatenate along first dimension)
  Constant : Constant  Value=Tw  VectorParams1D=off  SampleTime=-1
  Display : Display
  Edgewise_BM : Subsystem
  Flapwise_BM : Subsystem
  Gain1 : Gain  Gain=180/pi
  Lift/Drag : Subsystem
  LookUp_Table : Subsystem
  Only at root : Display
  Pitch : Constant
  Rotor Local radius : Constant  Value=r
  Rotor Speed : Constant  Value=14.9  VectorParams1D=off
  Scope1 : Scope  NumInputPorts=2
  Simulink-PS Converter : nesl_utility/Simulink-PS Converter  PhysicalDomain=network_engine_domain  SubClassName=ps_input  LeftPortType=input  RightPortType=output  PseudoPeriodic=off  Frequencies=[]  NoiseDistribution=none  NoiseParameters=[]  Unit=1  AffineConversion=off  FilteringAndDerivatives=provide  SimscapeFilterOrder=1  InputFilterTimeConstant=0.001  UdotUserProvided=0
  Sum : Sum  Inputs=|+-
  Sum2 : Sum  Inputs=|++
  To Workspace : ToWorkspace  VariableName=Flap_BM  SampleTime=-1
      settings: Save2DSignal=2-D array (concatenate along first dimension)
  Torque : Subsystem
  Twist : Constant  Commented=on  Value=T
  Wind angle : Subsystem
  Wind_Model : Subsystem
  AeroDy_Torque : PMIOPort  Side=Right
  tag scope: D=global, c=global
  wires:
  Rotor Local radius/1 -> Edgewise_BM/1(x), Flapwise_BM/1(x), Torque/3(r), Wind angle/3(r)
  Sum/1 -> LookUp_Table/1(AOA), AOA/1
  Lift/Drag/1(c) -> [c]
  Edgewise_BM/1(Edge_BM) -> Only at root/1
  Lift/Drag/3(D) -> [D]
  Wind_Model/1(Wind Speed V) -> Flapwise_BM/2(Wind Speed V), Scope1/1, Wind angle/1(V)  "Wind Speed V"
  LookUp_Table/1(Cl) -> Lift/Drag/2(Cl)
  LookUp_Table/4(Cd) -> Lift/Drag/5(Cd)
  LookUp_Table/3(Cl3) -> Lift/Drag/4(Cl3)
  LookUp_Table/2(Cl2) -> Lift/Drag/3(Cl2)
  Lift/Drag/2(dL) -> Torque/1(dL)
  Pitch/1 -> Sum2/2
  Wind angle/2(Vrc) -> Lift/Drag/1(Vr)
  Constant/1 -> Sum2/1
  Sum2/1 -> Sum/2
  LookUp_Table/6(Cd3) -> Lift/Drag/8(Cd3)
  Torque/1(Torq) -> Scope1/2, Simulink-PS Converter/1, Display/1  "Spinning Moment"
  Lift/Drag/4(dD) -> Torque/2(dD)
  Wind angle/1(FAc) -> Lift/Drag/6(FA in rad), Gain1/1
  Flapwise_BM/1(BM_Flap) -> To Workspace/1
  Rotor Speed/1 -> Wind angle/2(w)
  LookUp_Table/5(Cd2) -> Lift/Drag/7(Cd2)
  Gain1/1 -> Sum/1  "FA in deg"
  connections:
  Simulink-PS Converter/RConn1 -- AeroDy_Torque/RConn1

== system V90_2MW_TurbineModel_26_11_2021/Subsystem1/Edgewise_BM ==
  note: This Matlab Fcn gives Edgewise BM only at root. To calculate its variation along the Blade length, we need Mass/blade as UDL
  x : Inport
  MATLAB Function : MATLAB Function  TreatAsAtomicUnit=on
  Edge_BM : Outport
  wires:
  x/1 -> MATLAB Function/1(x)
  MATLAB Function/1(Edge_BM) -> Edge_BM/1

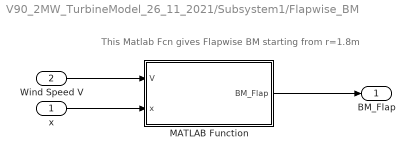
== system V90_2MW_TurbineModel_26_11_2021/Subsystem1/Flapwise_BM ==
  note: This Matlab Fcn gives Flapwise BM starting from r=1.8m
  x : Inport
  Wind Speed V : Inport  Port=2
  MATLAB Function : MATLAB Function  TreatAsAtomicUnit=on
  BM_Flap : Outport
  wires:
  MATLAB Function/1(BM_Flap) -> BM_Flap/1
  x/1 -> MATLAB Function/2(x)
  Wind Speed V/1 -> MATLAB Function/1(V)

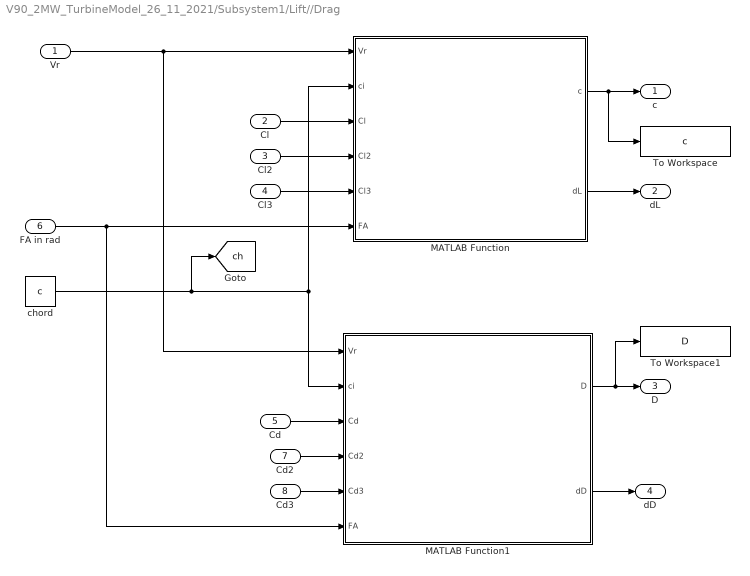
== system V90_2MW_TurbineModel_26_11_2021/Subsystem1/Lift//Drag ==
  Vr : Inport
  Cl : Inport  Port=2
  Cl2 : Inport  Port=3
  Cl3 : Inport  Port=4
  Cd : Inport  Port=5
  FA in rad : Inport  Port=6
  Cd2 : Inport  Port=7
  Cd3 : Inport  Port=8
  MATLAB Function : MATLAB Function  TreatAsAtomicUnit=on
  MATLAB Function1 : MATLAB Function  TreatAsAtomicUnit=on
  To Workspace : ToWorkspace  VariableName=c  SampleTime=-1
      settings: Save2DSignal=2-D array (concatenate along first dimension)
  To Workspace1 : ToWorkspace  VariableName=D  SampleTime=-1
      settings: Save2DSignal=2-D array (concatenate along first dimension)
  chord : Constant  Value=c
  c : Outport
  dL : Outport  Port=2
  D : Outport  Port=3
  dD : Outport  Port=4
  tag scope: ch=global
  wires:
  Cl2/1 -> MATLAB Function/4(Cl2)
  Cl/1 -> MATLAB Function/3(Cl)
  FA in rad/1 -> MATLAB Function1/6(FA), MATLAB Function/6(FA)
  Cd3/1 -> MATLAB Function1/5(Cd3)
  chord/1 -> MATLAB Function1/2(ci), MATLAB Function/2(ci), [ch]
  MATLAB Function/2(dL) -> dL/1
  Vr/1 -> MATLAB Function1/1(Vr), MATLAB Function/1(Vr)
  Cd2/1 -> MATLAB Function1/4(Cd2)
  Cl3/1 -> MATLAB Function/5(Cl3)
  Cd/1 -> MATLAB Function1/3(Cd)
  MATLAB Function1/2(dD) -> dD/1
  MATLAB Function1/1(D) -> To Workspace1/1, D/1
  MATLAB Function/1(c) -> To Workspace/1, c/1

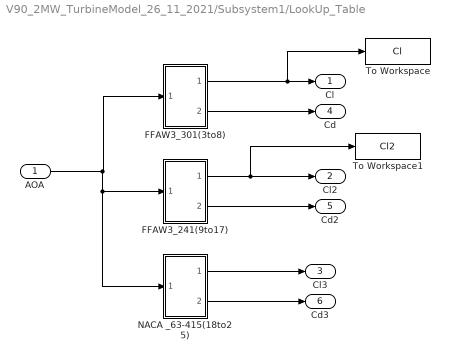
== system V90_2MW_TurbineModel_26_11_2021/Subsystem1/LookUp_Table ==
  AOA : Inport
  FFAW3_241(9to17) : Subsystem
  FFAW3_301(3to8) : Subsystem
  NACA _63-415(18to25) : Subsystem
  To Workspace : ToWorkspace  VariableName=Cl  SampleTime=-1
      settings: Save2DSignal=2-D array (concatenate along first dimension)
  To Workspace1 : ToWorkspace  VariableName=Cl2  SampleTime=-1
      settings: Save2DSignal=2-D array (concatenate along first dimension)
  Cl : Outport
  Cl2 : Outport  Port=2
  Cl3 : Outport  Port=3
  Cd : Outport  Port=4
  Cd2 : Outport  Port=5
  Cd3 : Outport  Port=6
  wires:
  FFAW3_301(3to8)/2(Output1) -> Cd/1
  AOA/1 -> NACA _63-415(18to25)/1(AOA), FFAW3_241(9to17)/1(AOA), FFAW3_301(3to8)/1(In1)
  FFAW3_301(3to8)/1(Output) -> To Workspace/1, Cl/1
  FFAW3_241(9to17)/1(Output) -> To Workspace1/1, Cl2/1
  FFAW3_241(9to17)/2(Output1) -> Cd2/1
  NACA _63-415(18to25)/1(Output) -> Cl3/1
  NACA _63-415(18to25)/2(Output1) -> Cd3/1

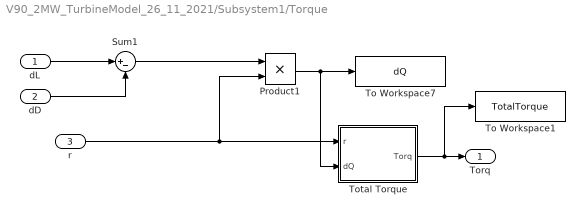
== system V90_2MW_TurbineModel_26_11_2021/Subsystem1/Torque ==
  dL : Inport
  dD : Inport  Port=2
  r : Inport  Port=3
  Product1 : Product
  Sum1 : Sum  Inputs=|+-
  To Workspace1 : ToWorkspace  VariableName=TotalTorque  SampleTime=-1
      settings: Save2DSignal=2-D array (concatenate along first dimension)
  To Workspace7 : ToWorkspace  VariableName=dQ  SampleTime=-1
      settings: Save2DSignal=2-D array (concatenate along first dimension)
  Total Torque : MATLAB Function  TreatAsAtomicUnit=on
  Torq : Outport
  wires:
  r/1 -> Product1/2, Total Torque/1(r)
  Product1/1 -> To Workspace7/1, Total Torque/2(dQ)
  dD/1 -> Sum1/2
  Total Torque/1(Torq) -> To Workspace1/1, Torq/1
  Sum1/1 -> Product1/1
  dL/1 -> Sum1/1

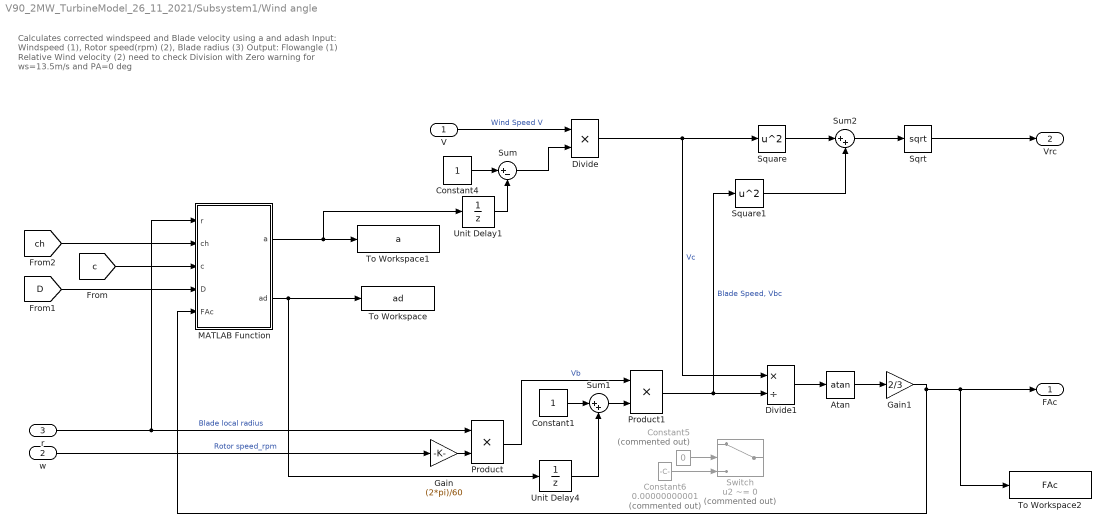
== system V90_2MW_TurbineModel_26_11_2021/Subsystem1/Wind angle ==
  note: Calculates corrected windspeed and Blade velocity using a and adash
      |
      | Input:
      | Windspeed (1),
      | Rotor speed(rpm) (2),
      | Blade radius (3)
      |
      | Output:
      | Flowangle (1)
      | Relative Wind velocity (2)
      |
      | need to check Division with Zero warning for ws=13.5m/s and PA=0 deg
  V : Inport
  w : Inport  Port=2
  r : Inport  Port=3
  Atan : Trigonometry  Operator=atan
  Constant1 : Constant
  Constant4 : Constant
  Constant5 : Constant  Commented=on  Value=0
  Constant6 : Constant  Commented=on  Value=0.00000000001
  Divide : Product  Inputs=**
  Divide1 : Product  Inputs=*/
  Gain : Gain  Gain=(2*pi)/60
  Gain1 : Gain  Gain=2/3
  MATLAB Function : MATLAB Function  TreatAsAtomicUnit=on
  Product : Product
  Product1 : Product
  Sqrt : Sqrt  SaturateOnIntegerOverflow=on
  Square : Math  Operator=square  SaturateOnIntegerOverflow=on
  Square1 : Math  Operator=square  SaturateOnIntegerOverflow=on
  Sum : Sum  Inputs=|+-
  Sum1 : Sum  Inputs=|++
  Sum2 : Sum  Inputs=|++
  Switch : Switch  Commented=on  Criteria=u2 ~= 0
  To Workspace : ToWorkspace  VariableName=ad  SampleTime=-1
      settings: Save2DSignal=2-D array (concatenate along first dimension)
  To Workspace1 : ToWorkspace  VariableName=a  SampleTime=-1
      settings: Save2DSignal=2-D array (concatenate along first dimension)
  To Workspace2 : ToWorkspace  VariableName=FAc  SampleTime=-1
      settings: Save2DSignal=2-D array (concatenate along first dimension)
  Unit Delay1 : UnitDelay  SampleTime=-1  HasFrameUpgradeWarning=on
  Unit Delay4 : UnitDelay  SampleTime=-1  HasFrameUpgradeWarning=on
  FAc : Outport
  Vrc : Outport  Port=2
  wires:
  Gain/1 -> Product/2
  Sum/1 -> Divide/2
  Constant4/1 -> Sum/1
  Divide1/1 -> Atan/1
  w/1 -> Gain/1  "Rotor speed_rpm"
  Constant1/1 -> Sum1/1
  Sum1/1 -> Product1/2
  r/1 -> Product/1, MATLAB Function/1(r)  "Blade local radius"
  Square/1 -> Sum2/1
  Square1/1 -> Sum2/2
  Sum2/1 -> Sqrt/1
  Sqrt/1 -> Vrc/1
  [ch] -> MATLAB Function/2(ch)
  MATLAB Function/2(ad) -> Unit Delay4/1, To Workspace/1
  MATLAB Function/1(a) -> Unit Delay1/1, To Workspace1/1
  V/1 -> Divide/1  "Wind Speed V"
  Divide/1 -> Square/1, Divide1/1  "Vc"
  Product/1 -> Product1/1  "Vb"
  Product1/1 -> Divide1/2, Square1/1  "Blade Speed, Vbc"
  Atan/1 -> Gain1/1
  Gain1/1 -> To Workspace2/1, FAc/1, MATLAB Function/5(FAc)
  Unit Delay1/1 -> Sum/2
  Unit Delay4/1 -> Sum1/2
  [D] -> MATLAB Function/4(D)
  [c] -> MATLAB Function/3(c)
  Constant5/1 -> Switch/2
  Constant6/1 -> Switch/3

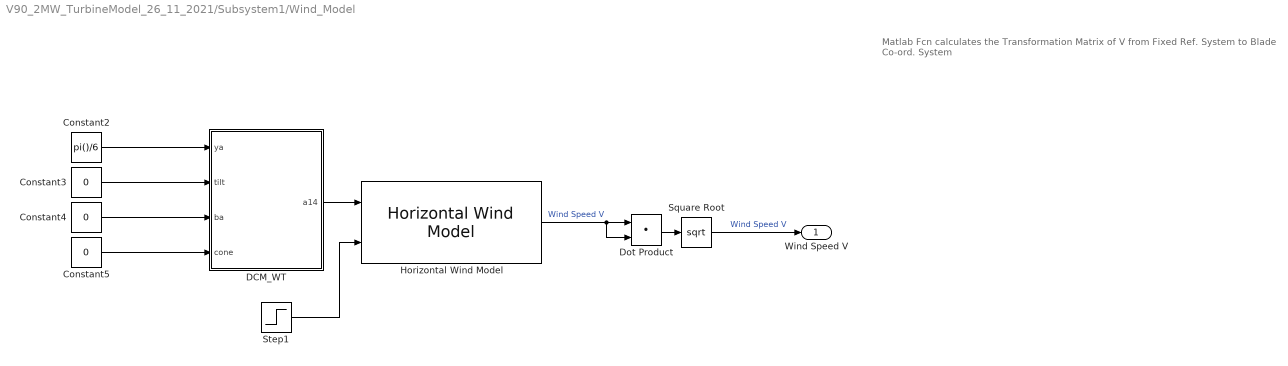
== system V90_2MW_TurbineModel_26_11_2021/Subsystem1/Wind_Model ==
  note: Matlab Fcn calculates the Transformation Matrix of V
      | from Fixed Ref. System to Blade Co-ord. System
  Constant2 : Constant  Value=pi()/6
  Constant3 : Constant  Value=0
  Constant4 : Constant  Value=0
  Constant5 : Constant  Value=0
  DCM_WT : MATLAB Function  TreatAsAtomicUnit=on
  Dot Product : DotProduct  InputSameDT=on  OutDataTypeStr=Inherit: Inherit via internal rule
  Horizontal Wind Model : aerolibwind2/Horizontal Wind Model  units=Metric (MKS)  Vw_source=External  Vwind=13.5  W_source=Internal  Wdeg=30
      settings: SourceProductBaseCode=AE
  Square Root : Sqrt  SaturateOnIntegerOverflow=on
  Step1 : Step  Time=0  After=13.5  SampleTime=0
  Wind Speed V : Outport
  wires:
  Step1/1 -> Horizontal Wind Model/2
  Square Root/1 -> Wind Speed V/1  "Wind Speed V"
  Horizontal Wind Model/1 -> Dot Product/2, Dot Product/1  "Wind Speed V"
  Dot Product/1 -> Square Root/1
  Constant5/1 -> DCM_WT/4(cone)
  DCM_WT/1(a14) -> Horizontal Wind Model/1
  Constant4/1 -> DCM_WT/3(ba)
  Constant2/1 -> DCM_WT/1(ya)
  Constant3/1 -> DCM_WT/2(tilt)

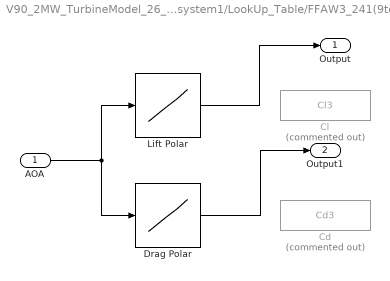
== system V90_2MW_TurbineModel_26_11_2021/Subsystem1/LookUp_Table/FFAW3_241(9to17) ==
  AOA : Inport
  Cd : ToWorkspace  Commented=on  VariableName=Cd3  SampleTime=-1
      settings: Save2DSignal=2-D array (concatenate along first dimension)
  Cl : ToWorkspace  Commented=on  VariableName=Cl3  SampleTime=-1
      settings: Save2DSignal=2-D array (concatenate along first dimension)
  Drag Polar : Lookup_n-D  NumberOfTableDimensions=1  BreakpointsForDimension1=|  Table=|  InternalRulePriority=Speed  RndMeth=Simplest  InputSameDT=on
      BreakpointsForDimension1=|
      | [-4.66442953
      | -3.951342282
      | -3.36409396
      | -2.609060403
      | -1.895973154
      | -1.266778523
      | -0.511744966
      | 0.033557047
      | 0.830536913
      | 1.543624161
      | 2.088926174
      | 2.718120805
      | 3.55704698
      | 4.270134228
      | 5.067114094
      | 6.031879195
      | 6.954697987
      | 7.583892617
      | 8.296979866
      | 8.968120805
      | 9.639261745
      | 10.26845638
      | 11.23322148
      | 11.90436242
      | 12.44966443
      | 12.95302013
      | 13.70805369
      | 14.2533557
      | 14.75671141
      | 15.26006711
      | 15.76342282
      | 16.01510067]
      Table=|
      | [0.010843373
      | 0.010240964
      | 0.009939759
      | 0.010240964
      | 0.009638554
      | 0.009939759
      | 0.009337349
      | 0.009939759
      | 0.009939759
      | 0.010542169
      | 0.010542169
      | 0.011144578
      | 0.011144578
      | 0.011746988
      | 0.012349398
      | 0.012650602
      | 0.014156627
      | 0.014457831
      | 0.014759036
      | 0.016566265
      | 0.017168675
      | 0.017771084
      | 0.020180723
      | 0.021385542
      | 0.022289157
      | 0.023192771
      | 0.026204819
      | 0.028012048
      | 0.031024096
      | 0.034337349
      | 0.039457831
      | 0.041566265]
  Lift Polar : Lookup_n-D  NumberOfTableDimensions=1  BreakpointsForDimension1=|  Table=|  InternalRulePriority=Speed  RndMeth=Simplest  InputSameDT=on
      BreakpointsForDimension1=|
      | [0.165837479
      | 0.870646766
      | 1.451077944
      | 2.031509121
      | 2.529021559
      | 3.109452736
      | 3.565505804
      | 4.104477612
      | 4.60199005
      | 5.016583748
      | 5.679933665
      | 6.343283582
      | 6.92371476
      | 7.587064677
      | 8.084577114
      | 8.830845771
      | 9.577114428
      | 9.950248756
      | 10.61359867
      | 11.35986733
      | 12.10613599
      | 12.89386401
      | 13.64013267
      | 14.51077944
      | 15.46434494
      | 16.12769486
      | 16.83250415
      | 17.66169154
      | 18.44941957
      | 19.32006633
      | 20.02487562
      | 20.77114428
      | 21.51741294
      | 22.30514096
      | 22.96849088
      | 23.79767828
      | 24.25373134
      | 24.66832504]
      Table=|
      | [0.238095238
      | 0.285714286
      | 0.357142857
      | 0.416666667
      | 0.5
      | 0.55952381
      | 0.607142857
      | 0.654761905
      | 0.720238095
      | 0.785714286
      | 0.845238095
      | 0.922619048
      | 1
      | 1.035714286
      | 1.107142857
      | 1.166666667
      | 1.244047619
      | 1.297619048
      | 1.357142857
      | 1.398809524
      | 1.44047619
      | 1.517857143
      | 1.523809524
      | 1.458333333
      | 1.43452381
      | 1.422619048
      | 1.416666667
      | 1.410714286
      | 1.392857143
      | 1.380952381
      | 1.357142857
      | 1.345238095
      | 1.30952381
      | 1.297619048
      | 1.279761905
      | 1.279761905
      | 1.261904762
      | 1.214285714]
  Output : Outport
  Output1 : Outport  Port=2
  wires:
  AOA/1 -> Drag Polar/1, Lift Polar/1
  Drag Polar/1 -> Output1/1
  Lift Polar/1 -> Output/1
